simulink model "MSD_final"  (R2021a)
settings: Solver=VariableStepAuto  StartTime=0.0  StopTime=10.0  RelTol=1e-3
settings Model: Creator=rachelj  LastModifiedBy=smuckati
settings SolverCC: AlgebraicLoopSolver=TrustRegion
settings DebuggingCC: SFMachineParentedDataDiag=warning  ArithmeticOperatorsInVariantConditions=warning
settings SFSimCC: CustomCodeUndefinedFunction=UseInterfaceOnly

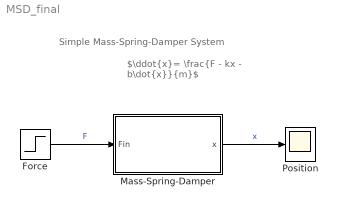
== system MSD_final ==
  note: Simple Mass-Spring-Damper System
  note: $\ddot{x}= \frac{F - kx - b\dot{x}}{m}$
  Force : Step  SampleTime=0
  Mass-Spring-Damper : Subsystem  mask{k=50, b=0, m=10}
      mask prompts: k "Stiffness ="; b "Damping ="; m "Mass ="
      mask Display: image('$imagefile'); % Use "Edit Image" on toolstrip to change.
  Position : Scope
  wires:
  Force/1 -> Mass-Spring-Damper/1(Fin)  "F"
  Mass-Spring-Damper/1(x) -> Position/1  "x"

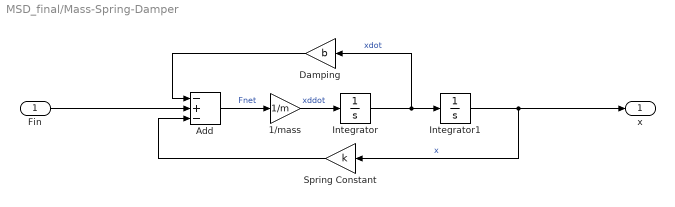
== system MSD_final/Mass-Spring-Damper ==
  Fin : Inport
  1/mass : Gain  Gain=1/m
  Add : Sum  Inputs=-+-
  Damping : Gain  Gain=b
  Integrator : Integrator
  Integrator1 : Integrator
  Spring Constant : Gain  Gain=k
  x : Outport  VectorParamsAs1DForOutWhenUnconnected=off
  wires:
  Add/1 -> 1/mass/1  "Fnet"
  Integrator1/1 -> x/1, Spring Constant/1  "x"
  1/mass/1 -> Integrator/1  "xddot"
  Fin/1 -> Add/2
  Integrator/1 -> Damping/1, Integrator1/1  "xdot"
  Damping/1 -> Add/1
  Spring Constant/1 -> Add/3
